simulink model "DBL_Master_Runner"  (R2020b)
settings: configuration reference "VLS_Standard_Configuration" (kept outside this file)
settings Model: DataDictionary=DBL_Master_DD.sldd  EnableAccessToBaseWorkspace=off  Creator=mteama  LastModifiedBy=ahashem
settings ConfigSetRef: SourceName=VLS_Standard_Configuration

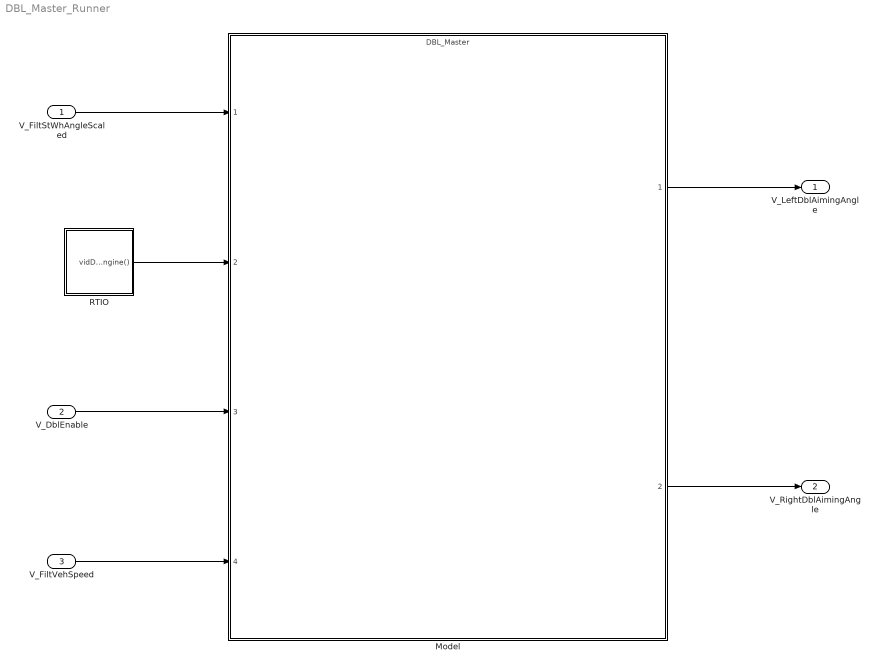
== system DBL_Master_Runner ==
  V_FiltStWhAngleScaled : Inport  OutDataTypeStr=fixdt(1,16,0.1,0)  PortDimensions=1
  V_DblEnable : Inport  Port=2  OutDataTypeStr=boolean  PortDimensions=1
  V_FiltVehSpeed : Inport  Port=3  OutDataTypeStr=fixdt(0,16,0.1,0)  PortDimensions=1
  Model : ModelReference  ModelNameDialog=DBL_Master.slx  SimulationMode=Normal  ScheduleRates=on  ModelReferenceVersion=7.87
  RTIO : Stateflow chart  TreatAsAtomicUnit=on  SystemSampleTime=0.02
  V_LeftDblAimingAngle : Outport  PortDimensions=1
  V_RightDblAimingAngle : Outport  Port=2  PortDimensions=1
  wires:
  RTIO/1(vidDBLM_Engine()) -> Model/2
  V_FiltStWhAngleScaled/1 -> Model/1
  Model/1 -> V_LeftDblAimingAngle/1
  V_DblEnable/1 -> Model/3
  V_FiltVehSpeed/1 -> Model/4
  Model/2 -> V_RightDblAimingAngle/1

== stateflow chart DBL_Master_Runner/RTIO ==
  state Schedule
    on every(1,tick):
    send(vidDBLM_Engine)
  (default) -> Schedule
  events: vidDBLM_Engine output FUNCTION_CALL_EVENT
